simulink model "MalhaExternaSimplificadaR2018b"  (R2018b)
settings: Solver=ode23s  StartTime=0.0  StopTime=10.0  RelTol=1e-3
values from neighbouring files (symbols this model uses):
  dt = 0.001    [Main_Malha_Externa.m]    (also in Main_Malha_Externa_referencia.m; main.m; main_malha_interna.m; otimiza_Dir.m)
  x = fmincon(@otimiza_PIDF,x,[],[],[],[],[0 0 0 0],[inf inf inf inf],@QQQ,options)    [Main_Malha_Externa.m]    (also in Main_Malha_Externa_referencia.m = fmincon(@otimiza_PIDF_referencia,x,[],[],[],[],[0 0 0 0],[in; main.m = fmincon(@otimiza_Esq,x,[],[],[],[],[0 0 0],[inf inf 1400],@Q; main_malha_interna.m = fmincon(@otimiza_Esq,x,[],[],[],[],[0 0 0],[inf inf 1400],@Q; otimiza_Dir.m = X)
settings Model: Creator=lucas  LastModifiedBy=vitor
settings DataIOCC: ReturnWorkspaceOutputs=on
settings DebuggingCC: SFMachineParentedDataDiag=error

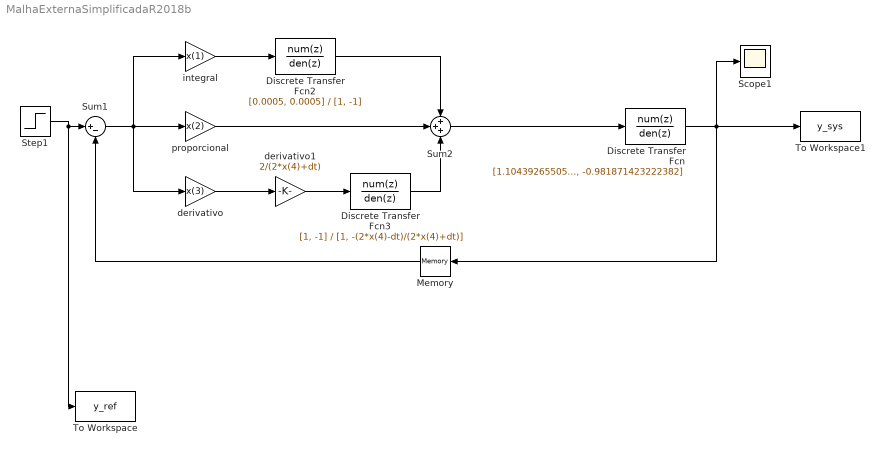
== system MalhaExternaSimplificadaR2018b ==
  Discrete Transfer Fcn : DiscreteTransferFcn  Numerator=[1.104392655054829e-08, 3.313177965164485e-08, 3.313177965164485e-08, 1.104392655054829e-08]  Denominator=[1, -2.981694681338594, 2.963566104560976, -0.981871423222382]
  Discrete Transfer Fcn2 : DiscreteTransferFcn  Numerator=[0.0005, 0.0005]  Denominator=[1, -1]
  Discrete Transfer Fcn3 : DiscreteTransferFcn  Numerator=[1, -1]  Denominator=[1, -(2*x(4)-dt)/(2*x(4)+dt)]  SampleTime=0.001
  Memory : Memory  InheritSampleTime=on
  Scope1 : Scope
  Step1 : Step  Time=0  After=0.3  SampleTime=0.001
  Sum1 : Sum  Inputs=|+-
  Sum2 : Sum  Inputs=+++
  To Workspace : ToWorkspace  VariableName=y_ref  SampleTime=-1
  To Workspace1 : ToWorkspace  VariableName=y_sys  SampleTime=-1
  derivativo : Gain  Gain=x(3)
  derivativo1 : Gain  Gain=2/(2*x(4)+dt)
  integral : Gain  Gain=x(1)
  proporcional : Gain  Gain=x(2)
  wires:
  Step1/1 -> To Workspace/1, Sum1/1
  Sum2/1 -> Discrete Transfer Fcn/1
  Discrete Transfer Fcn/1 -> To Workspace1/1, Memory/1, Scope1/1
  Memory/1 -> Sum1/2
  Discrete Transfer Fcn2/1 -> Sum2/1
  Discrete Transfer Fcn3/1 -> Sum2/3
  integral/1 -> Discrete Transfer Fcn2/1
  proporcional/1 -> Sum2/2
  derivativo/1 -> derivativo1/1
  derivativo1/1 -> Discrete Transfer Fcn3/1
  Sum1/1 -> derivativo/1, integral/1, proporcional/1
